simulink model "Coupled_drives_task2a"  (R2020a)
settings: Solver=VariableStepAuto  StartTime=0.0  StopTime=200  RelTol=1e-3
settings Model: Creator=nbl  LastModifiedBy=philipgutierrez
settings DataIOCC: ReturnWorkspaceOutputs=off
settings DebuggingCC: PregeneratedLibrarySubsystemCodeDiagnostic=none  ArithmeticOperatorsInVariantConditions=warning
settings SFSimCC: SimUseLocalCustomCode=off  CustomCodeUndefinedFunction=UseInterfaceOnly
settings RTWCC: RTWUseLocalCustomCode=off

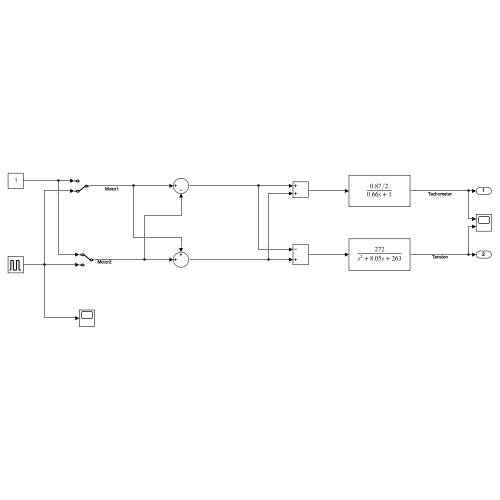
[thumbnail: Simulink's stored preview of the top-level diagram]
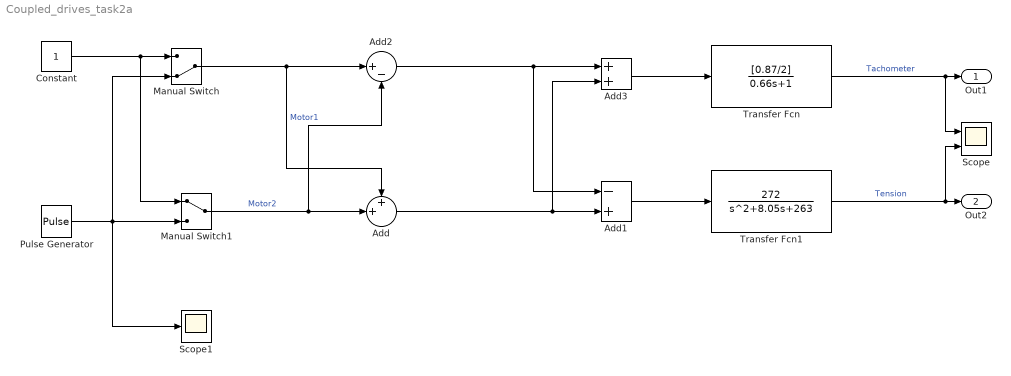
== system Coupled_drives_task2a ==
  Add : Sum  Inputs=++|
  Add1 : Sum  Inputs=-+
  Add2 : Sum  Inputs=|+-
  Add3 : Sum  Inputs=2
  Constant : Constant
  Manual Switch : ManualSwitch  CurrentSetting=0
  Manual Switch1 : ManualSwitch
  Pulse Generator : DiscretePulseGenerator  PulseType=Time based  Period=50  PulseWidth=50
  Scope : Scope  NumInputPorts=2
  Scope1 : Scope
  Transfer Fcn : TransferFcn  Numerator=[0.87/2]  Denominator=[0.66 1]
  Transfer Fcn1 : TransferFcn  Numerator=[272]  Denominator=[1 8.05 263]
  Out1 : Outport  VectorParamsAs1DForOutWhenUnconnected=off
  Out2 : Outport  Port=2  VectorParamsAs1DForOutWhenUnconnected=off
  wires:
  Add3/1 -> Transfer Fcn/1
  Add1/1 -> Transfer Fcn1/1
  Transfer Fcn/1 -> Out1/1, Scope/1  "Tachometer"
  Transfer Fcn1/1 -> Out2/1, Scope/2  "Tension"
  Add/1 -> Add3/2, Add1/2
  Add2/1 -> Add3/1, Add1/1
  Manual Switch/1 -> Add/1, Add2/1  "Motor1"
  Constant/1 -> Manual Switch1/1, Manual Switch/1
  Manual Switch1/1 -> Add2/2, Add/2  "Motor2"
  Pulse Generator/1 -> Scope1/1, Manual Switch/2, Manual Switch1/2
